simulink model "model ciężarka na sprężynie"  (R2025b)
settings: Solver=ode23  StartTime=0.0  StopTime=2  RelTol=1e-3
settings Model: Creator=Student  LastModifiedBy=Student

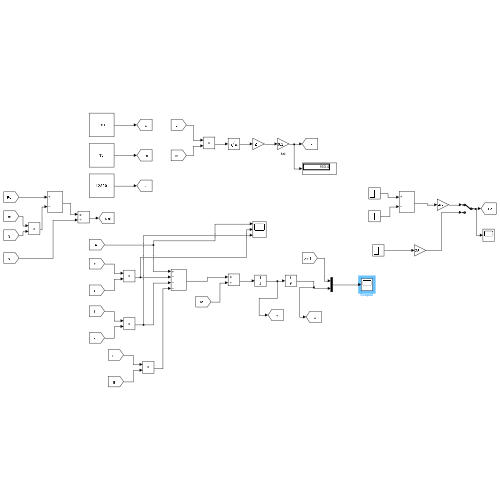
[thumbnail: Simulink's stored preview of the top-level diagram]
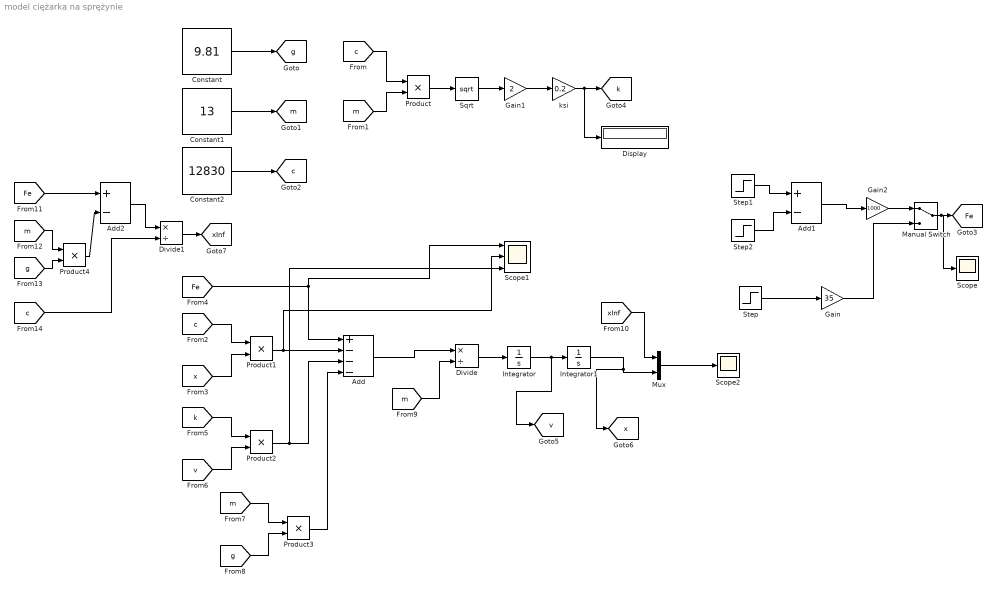
== system model ciężarka na sprężynie ==
  Add : Sum  Inputs=+---
  Add1 : Sum  Inputs=+-
  Add2 : Sum  Inputs=+-
  Constant : Constant  Value=9.81
  Constant1 : Constant  Value=13
  Constant2 : Constant  Value=12830
  Display : Display
  Divide : Product  Inputs=*/
  Divide1 : Product  Inputs=*/
  Gain : Gain  Gain=35
  Gain1 : Gain  Gain=2
  Gain2 : Gain  Gain=1000
  Integrator : Integrator
  Integrator1 : Integrator
  Manual Switch : ManualSwitch
  Mux : Mux  Inputs=2
  Product{,1..4} (5 alike) : Product
  Scope : Scope
      settings: ActiveDisplayYMinimum=-1  ActiveDisplayYMaximum=1
  Scope1 : Scope  NumInputPorts=3
      settings: ActiveDisplayYMinimum=-4.3749999999999991  ActiveDisplayYMaximum=39.375
  Scope2 : Scope
      settings: ActiveDisplayYMinimum=-0.025487629352462356  ActiveDisplayYMaximum=0.078390112449918517  DataLoggingVariableName=ScopeData2
  Sqrt : Sqrt
  Step : Step  SampleTime=0
  Step1 : Step  SampleTime=0
  Step2 : Step  Time=1.001  SampleTime=0
  ksi : Gain  Gain=0.2
  tag scope: Fe=global, c=global, g=global, k=global, m=global, v=global, x=global, xInf=global
  wires:
  Constant/1 -> [g]
  Constant1/1 -> [m]
  Constant2/1 -> [c]
  Step/1 -> Gain/1
  Gain/1 -> Manual Switch/2
  [c] -> Product/1
  [m] -> Product/2
  Product/1 -> Sqrt/1
  Sqrt/1 -> Gain1/1
  Gain1/1 -> ksi/1
  ksi/1 -> Display/1, [k]
  [c] -> Product1/1
  [x] -> Product1/2
  [v] -> Product2/2
  [k] -> Product2/1
  [m] -> Product3/1
  [g] -> Product3/2
  Product1/1 -> Scope1/2, Add/2
  Product2/1 -> Scope1/3, Add/3
  Product3/1 -> Add/4
  [Fe] -> Add/1, Scope1/1
  Add/1 -> Divide/1
  [m] -> Divide/2
  Divide/1 -> Integrator/1
  Integrator/1 -> [v], Integrator1/1
  Integrator1/1 -> [x], Mux/2
  Mux/1 -> Scope2/1
  Step1/1 -> Add1/1
  Step2/1 -> Add1/2
  Add1/1 -> Gain2/1
  Gain2/1 -> Manual Switch/1
  Manual Switch/1 -> Scope/1, [Fe]
  [m] -> Product4/1
  [g] -> Product4/2
  Product4/1 -> Add2/2
  [Fe] -> Add2/1
  Divide1/1 -> [xInf]
  Add2/1 -> Divide1/1
  [c] -> Divide1/2
  [xInf] -> Mux/1
